simulink model "Task1"  (R2022a)
settings: Solver=FixedStepAuto  StartTime=0.0  StopTime=20  FixedStep=0.0001  RelTol=1e-3
settings Model: Creator=Family  LastModifiedBy=Family

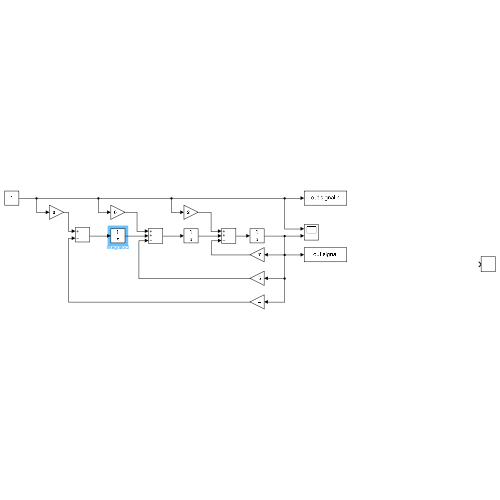
[thumbnail: Simulink's stored preview of the top-level diagram]
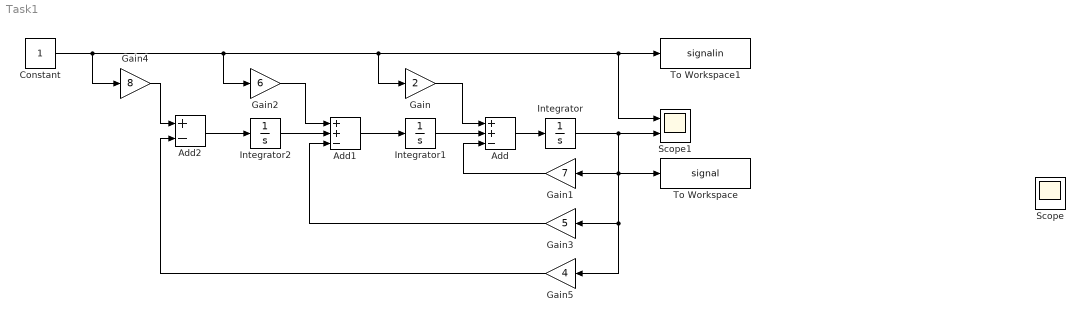
== system Task1 ==
  Add : Sum  Inputs=++-
  Add1 : Sum  Inputs=++-
  Add2 : Sum  Inputs=+-
  Constant : Constant  SampleTime=-1
  Gain : Gain  Gain=2
  Gain1 : Gain  Gain=7
  Gain2 : Gain  Gain=6
  Gain3 : Gain  Gain=5
  Gain4 : Gain  Gain=8
  Gain5 : Gain  Gain=4
  Integrator : Integrator
  Integrator1 : Integrator
  Integrator2 : Integrator
  Scope : Scope
  Scope1 : Scope  NumInputPorts=2
  To Workspace : ToWorkspace  VariableName=signal  SaveFormat=Timeseries  SampleTime=-1
  To Workspace1 : ToWorkspace  VariableName=signalin  SaveFormat=Timeseries  SampleTime=-1
  wires:
  Integrator/1 -> Scope1/2, To Workspace/1, Gain5/1, Gain3/1, Gain1/1
  Gain/1 -> Add/1
  Gain1/1 -> Add/3
  Integrator1/1 -> Add/2
  Add1/1 -> Integrator1/1
  Gain2/1 -> Add1/1
  Gain3/1 -> Add1/3
  Integrator2/1 -> Add1/2
  Add2/1 -> Integrator2/1
  Gain4/1 -> Add2/1
  Gain5/1 -> Add2/2
  Add/1 -> Integrator/1
  Constant/1 -> Scope1/1, To Workspace1/1, Gain/1, Gain2/1, Gain4/1
